simulink model "vaporizer"  (Simulink 7.8)
settings: Solver=ode45  StartTime=0.0  StopTime=20  RelTol=1e-3
settings Model: Creator=Max  LastModifiedBy=Max

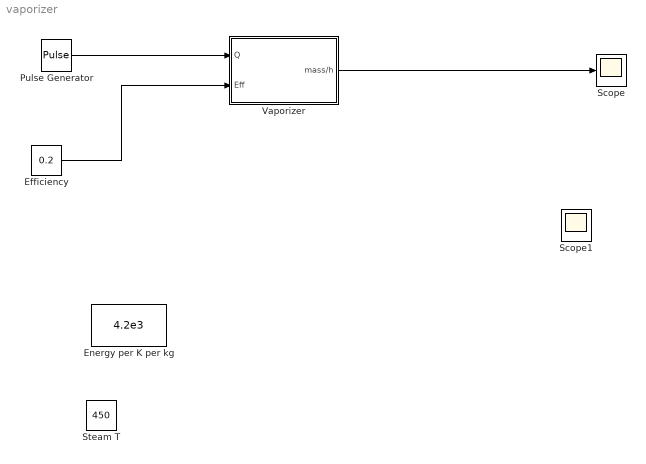
== system vaporizer ==
  Efficiency : Constant  Value=0.2
  Energy per K per kg : Constant  Value=4.2e3
  Pulse Generator : DiscretePulseGenerator  PulseType=Time based  Amplitude=2e9  Period=10  PulseWidth=50  PhaseDelay=1
  Scope : Scope
  Scope1 : Scope
  Steam T : Constant  Value=450
  Vaporizer : Subsystem  TreatAsAtomicUnit=on
  wires:
  Pulse Generator/1 -> Vaporizer/1(Q)
  Vaporizer/1(mass/h) -> Scope/1
  Efficiency/1 -> Vaporizer/2(Eff)

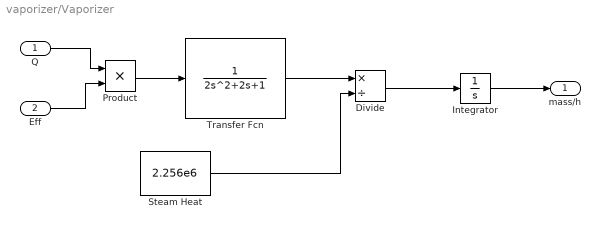
== system vaporizer/Vaporizer ==
  Q : Inport
  Eff : Inport  Port=2
  Divide : Product  Inputs=*/
  Integrator : Integrator
  Product : Product  RndMeth=Zero
  Steam Heat : Constant  Value=2.256e6
  Transfer Fcn : TransferFcn  Denominator=[2 2 1]
  mass/h : Outport
  wires:
  Steam Heat/1 -> Divide/2
  Transfer Fcn/1 -> Divide/1
  Divide/1 -> Integrator/1
  Product/1 -> Transfer Fcn/1
  Q/1 -> Product/1
  Eff/1 -> Product/2
  Integrator/1 -> mass/h/1
